simulink model "Actuator_Spring_Mass_Control_Design"  (R2018b)
settings: Solver=VariableStepAuto  StartTime=0.0  StopTime=10  RelTol=1e-3
model workspace: external: MATLAB File C:\Users\dmesenge\Documents\School\Modern Control Thoery\Project\ElectricMotorControl.m (data not in the file)
values from neighbouring files (symbols this model uses):
  A = [0 1         0 ... (first row only)    [Actuator_Spring_Mass_controller.m]
  As = [0     1 ... (first row only)    [Actuator_Spring_Mass_controller.m]
  B = [0 ... (first row only)    [Actuator_Spring_Mass_controller.m]
  Bs = [0 ... (first row only)    [Actuator_Spring_Mass_controller.m]
  C = [1   0   0]    [Actuator_Spring_Mass_controller.m]
  Cs = [k   0]    [Actuator_Spring_Mass_controller.m]
  D = 0    [Actuator_Spring_Mass_controller.m]
  Ds = 0    [Actuator_Spring_Mass_controller.m]
  K = lqi(motor_ss, Q, R)    [Actuator_Spring_Mass_controller.m]
  Ks = lqi(spring_ss, Qs, Rs)    [Actuator_Spring_Mass_controller.m]
  W = 0.05    [Actuator_Spring_Mass_controller.m]
undefined symbols (not defined in the file or in its folder): Continuous, Time
libraries: ctrlSharedLib x2
settings Model: Creator=dmesenge  LastModifiedBy=dmesenge

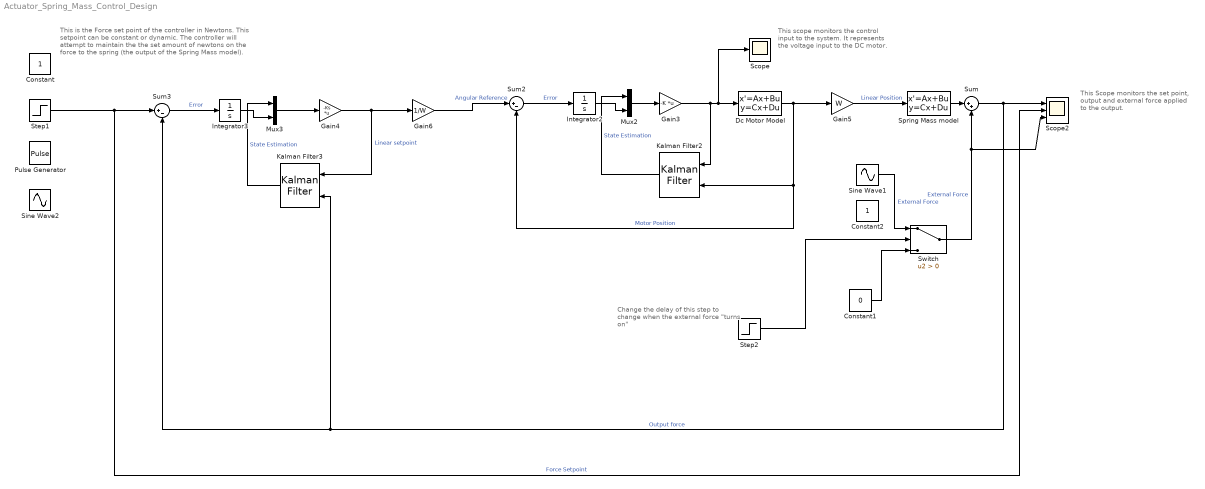
== system Actuator_Spring_Mass_Control_Design ==
  note: Change the delay of this step to change when the external force "turns on"
  note: This Scope monitors the set point, output and external force applied to the output.
  note: This scope monitors the control input to the system. It represents the voltage input to the DC motor.
  note: This is the Force set point of the controller in Newtons. This setpoint can be constant or dynamic. The controller will attempt to maintain the the set amount of newtons on the force to the spring (the output of the Spring Mass model).
  Constant : Constant
  Constant1 : Constant  Value=0
  Constant2 : Constant
  Dc Motor Model : StateSpace  A=A  B=B  C=C  D=D  InitialCondition=0
  Gain3 : Gain  Gain=-K  Multiplication=Matrix(K*u)
  Gain4 : Gain  Gain=-Ks  Multiplication=Matrix(K*u)
  Gain5 : Gain  Gain=W
  Gain6 : Gain  Gain=1/W
  Integrator2 : Integrator
  Integrator3 : Integrator
  Kalman Filter2 : ctrlSharedLib/Kalman Filter  TimeDomain=Continuous-Time  UseCurrentEstimator=on  ModelSource=LTI State-Space Variable  ModelSourceVariable=motor_ss  A=0.95  B=1  C=1  D=0  NumberOfStates=1  NumberOfInputs=1  NumberOfOutputs=1  InitialEstimateSource=Dialog  X0=0  P0=10  UseK=off  UseGH=off  NumberOfProcessNoiseInputs=1  G=1  TimeInvariantG=on  H=0  TimeInvariantH=on  Q=0.05  TimeInvariantQ=on  R=1  TimeInvariantR=on  N=0  TimeInvariantN=on  AddInputPort=on  AddEnablePort=off  OutputEstimatedY=off  OutputP=off  Ts=-1
      settings: SourceProductBaseCode=CT
  Kalman Filter3 : ctrlSharedLib/Kalman Filter  TimeDomain=Continuous-Time  UseCurrentEstimator=on  ModelSource=LTI State-Space Variable  ModelSourceVariable=spring_ss  A=0.95  B=1  C=1  D=0  NumberOfStates=1  NumberOfInputs=1  NumberOfOutputs=1  InitialEstimateSource=Dialog  X0=0  P0=10  UseK=off  UseGH=off  NumberOfProcessNoiseInputs=1  G=1  TimeInvariantG=on  H=0  TimeInvariantH=on  Q=0.05  TimeInvariantQ=on  R=1  TimeInvariantR=on  N=0  TimeInvariantN=on  AddInputPort=on  AddEnablePort=off  OutputEstimatedY=off  OutputP=off  Ts=-1
      settings: SourceProductBaseCode=CT
  Mux2 : Mux  Inputs=2
  Mux3 : Mux  Inputs=2
  Pulse Generator : DiscretePulseGenerator  PulseType=Time based  PulseWidth=50
  Scope : Scope
  Scope2 : Scope  NumInputPorts=3
  Sine Wave1 : Sin  SampleTime=0
  Sine Wave2 : Sin  SampleTime=0
  Spring Mass model : StateSpace  A=As  B=Bs  C=Cs  D=Ds  InitialCondition=0
  Step1 : Step  SampleTime=0
  Step2 : Step  SampleTime=5
  Sum : Sum  Inputs=|++
  Sum2 : Sum  Inputs=|+-
  Sum3 : Sum  Inputs=|+-
  Switch : Switch  Criteria=u2 > Threshold
  wires:
  Sum2/1 -> Integrator2/1  "Error"
  Gain3/1 -> Dc Motor Model/1, Scope/1, Kalman Filter2/1
  Integrator2/1 -> Mux2/2
  Kalman Filter2/1 -> Mux2/1  "State Estimation"
  Gain4/1 -> Gain6/1, Kalman Filter3/1  "Linear setpoint"
  Dc Motor Model/1 -> Sum2/2, Kalman Filter2/2, Gain5/1  "Motor Position"
  Mux2/1 -> Gain3/1
  Mux3/1 -> Gain4/1
  Sum/1 -> Kalman Filter3/2, Sum3/2, Scope2/1  "Output force"
  Sum3/1 -> Integrator3/1  "Error"
  Kalman Filter3/1 -> Mux3/1  "State Estimation"
  Integrator3/1 -> Mux3/2
  Step1/1 -> Sum3/1, Scope2/2  "Force Setpoint"
  Gain5/1 -> Spring Mass model/1  "Linear Position"
  Gain6/1 -> Sum2/1  "Angular Reference"
  Spring Mass model/1 -> Sum/1
  Switch/1 -> Sum/2, Scope2/3  "External Force"
  Step2/1 -> Switch/2
  Constant1/1 -> Switch/3
  Sine Wave1/1 -> Switch/1  "External Force"
